simulink model "h_bridge_cascaded_five_level_inverter"  (R2022b)
settings: Solver=ode3  StartTime=0.0  StopTime=0.045  FixedStep=1e-6  RelTol=1e-3  EnableMultiTasking=on
undefined symbols (not defined in the file): fc, fr, Ma, ph
libraries: spsIGBTDiodeLib x328, simulink x164, spsDCVoltageSourceLib x82, spsCurrentMeasurementLib x41, spsSeriesRLCBranchLib x41, spsVoltageMeasurementLib x41, spspowerguiLib x1
(part 3 of 3)

== system h_bridge_cascaded_five_level_inverter/Phase A33 ==
  100V : spsDCVoltageSourceLib/DC Voltage Source  Amplitude=100  Measurements=None
  100V1 : spsDCVoltageSourceLib/DC Voltage Source  Amplitude=100  Measurements=None
  NOT{,1..3} (4 alike) : Logic  Operator=NOT  AllPortsSameDT=off  OutDataTypeStr=boolean
  Relational Operator4 : RelationalOperator  OutDataTypeStr=boolean  InputSameDT=off
  Relational Operator5 : RelationalOperator  Operator=<=  OutDataTypeStr=boolean  InputSameDT=off
  Relational Operator6 : RelationalOperator  Operator=<=  OutDataTypeStr=boolean  InputSameDT=off
  Relational Operator7 : RelationalOperator  OutDataTypeStr=boolean  InputSameDT=off
  Repeating Sequence1 : simulink/Sources/Repeating Sequence  rep_seq_t=[0 0.00025 0.0005 0.00075 0.001]*(1/fr)*(1/fc)*(1/2)  rep_seq_y="[0 1 0 -1 0  ]"
  Repeating Sequence2 : simulink/Sources/Repeating Sequence  rep_seq_t=[0 0.00025 0.0005 0.00075 0.001]*(1/fr)*(1/fc)*(1/2)  rep_seq_y=[ 0 -1 0 1 0 ]
  Repeating Sequence5 : simulink/Sources/Repeating Sequence  rep_seq_t=[0 0.00025 0.0005 0.00075 0.001]*(1/fr)*(1/fc)*(1/2)  rep_seq_y=[1 0 -1 0 1]
  Repeating Sequence7 : simulink/Sources/Repeating Sequence  rep_seq_t=[0 0.00025 0.0005 0.00075 0.001]*(1/fr)*(1/fc)*(1/2)  rep_seq_y=[-1 0 1 0 -1]
  SW{1..8} (8 alike) : spsIGBTDiodeLib/IGBT//Diode  Ron=1e-3  Rs=1e5  Cs=inf  Measurements=on
  Sine Wave1 : Sin  Amplitude=Ma  Frequency=2*pi*fr  Phase=ph  SampleTime=0
  Sine Wave2 : Sin  Amplitude=Ma  Frequency=2*pi*fr  Phase=ph  SampleTime=0
  Va : PMIOPort  Tag=PMCPort  Side=Right
  N : PMIOPort  Tag=PMCPort  Port=2  Side=Right
  wires:
  Sine Wave2/1 -> Relational Operator4/1, Relational Operator6/1
  Repeating Sequence1/1 -> Relational Operator4/2
  Repeating Sequence2/1 -> Relational Operator6/2
  Relational Operator4/1 -> NOT/1, [S1]
  NOT/1 -> [S3]
  NOT1/1 -> [S4]
  Relational Operator6/1 -> [S2], NOT1/1
  Repeating Sequence7/1 -> Relational Operator7/2
  Repeating Sequence5/1 -> Relational Operator5/2
  Sine Wave1/1 -> Relational Operator7/1, Relational Operator5/1
  Relational Operator5/1 -> [S6], NOT3/1
  Relational Operator7/1 -> [S5], NOT2/1
  NOT2/1 -> [S7]
  NOT3/1 -> [S8]
  [S3] -> SW3/1
  [S6] -> SW6/1
  [S8] -> SW8/1
  [S1] -> SW1/1
  [S2] -> SW2/1
  [S4] -> SW4/1
  [S5] -> SW5/1
  connections:
  Va/RConn1 -- SW2/RConn1 -- SW4/LConn1
  SW4/RConn1 -- 100V/LConn1 -- SW3/RConn1
  SW8/RConn1 -- 100V1/LConn1 -- SW7/RConn1
  SW1/RConn1 -- SW3/LConn1 -- SW6/RConn1 -- SW8/LConn1
  SW5/LConn1 -- 100V1/RConn1 -- SW6/LConn1
  N/RConn1 -- SW5/RConn1 -- SW7/LConn1
  100V/RConn1 -- SW1/LConn1 -- SW2/LConn1

== system h_bridge_cascaded_five_level_inverter/Phase A34 ==
  100V : spsDCVoltageSourceLib/DC Voltage Source  Amplitude=100  Measurements=None
  100V1 : spsDCVoltageSourceLib/DC Voltage Source  Amplitude=100  Measurements=None
  NOT{,1..3} (4 alike) : Logic  Operator=NOT  AllPortsSameDT=off  OutDataTypeStr=boolean
  Relational Operator4 : RelationalOperator  OutDataTypeStr=boolean  InputSameDT=off
  Relational Operator5 : RelationalOperator  Operator=<=  OutDataTypeStr=boolean  InputSameDT=off
  Relational Operator6 : RelationalOperator  Operator=<=  OutDataTypeStr=boolean  InputSameDT=off
  Relational Operator7 : RelationalOperator  OutDataTypeStr=boolean  InputSameDT=off
  Repeating Sequence1 : simulink/Sources/Repeating Sequence  rep_seq_t=[0 0.00025 0.0005 0.00075 0.001]*(1/fr)*(1/fc)*(1/2)  rep_seq_y="[0 1 0 -1 0  ]"
  Repeating Sequence2 : simulink/Sources/Repeating Sequence  rep_seq_t=[0 0.00025 0.0005 0.00075 0.001]*(1/fr)*(1/fc)*(1/2)  rep_seq_y=[ 0 -1 0 1 0 ]
  Repeating Sequence5 : simulink/Sources/Repeating Sequence  rep_seq_t=[0 0.00025 0.0005 0.00075 0.001]*(1/fr)*(1/fc)*(1/2)  rep_seq_y=[1 0 -1 0 1]
  Repeating Sequence7 : simulink/Sources/Repeating Sequence  rep_seq_t=[0 0.00025 0.0005 0.00075 0.001]*(1/fr)*(1/fc)*(1/2)  rep_seq_y=[-1 0 1 0 -1]
  SW{1..8} (8 alike) : spsIGBTDiodeLib/IGBT//Diode  Ron=1e-3  Rs=1e5  Cs=inf  Measurements=on
  Sine Wave1 : Sin  Amplitude=Ma  Frequency=2*pi*fr  Phase=ph  SampleTime=0
  Sine Wave2 : Sin  Amplitude=Ma  Frequency=2*pi*fr  Phase=ph  SampleTime=0
  Va : PMIOPort  Tag=PMCPort  Side=Right
  N : PMIOPort  Tag=PMCPort  Port=2  Side=Right
  wires:
  Sine Wave2/1 -> Relational Operator4/1, Relational Operator6/1
  Repeating Sequence1/1 -> Relational Operator4/2
  Repeating Sequence2/1 -> Relational Operator6/2
  Relational Operator4/1 -> NOT/1, [S1]
  NOT/1 -> [S3]
  NOT1/1 -> [S4]
  Relational Operator6/1 -> [S2], NOT1/1
  Repeating Sequence7/1 -> Relational Operator7/2
  Repeating Sequence5/1 -> Relational Operator5/2
  Sine Wave1/1 -> Relational Operator7/1, Relational Operator5/1
  Relational Operator5/1 -> [S6], NOT3/1
  Relational Operator7/1 -> [S5], NOT2/1
  NOT2/1 -> [S7]
  NOT3/1 -> [S8]
  [S3] -> SW3/1
  [S6] -> SW6/1
  [S7] -> SW7/1
  [S8] -> SW8/1
  [S1] -> SW1/1
  [S2] -> SW2/1
  [S4] -> SW4/1
  connections:
  Va/RConn1 -- SW2/RConn1 -- SW4/LConn1
  SW4/RConn1 -- 100V/LConn1 -- SW3/RConn1
  SW8/RConn1 -- 100V1/LConn1 -- SW7/RConn1
  SW1/RConn1 -- SW3/LConn1 -- SW6/RConn1 -- SW8/LConn1
  SW5/LConn1 -- 100V1/RConn1 -- SW6/LConn1
  N/RConn1 -- SW5/RConn1 -- SW7/LConn1
  100V/RConn1 -- SW1/LConn1 -- SW2/LConn1

== system h_bridge_cascaded_five_level_inverter/Phase A42 ==
  100V : spsDCVoltageSourceLib/DC Voltage Source  Amplitude=100  Measurements=None
  100V1 : spsDCVoltageSourceLib/DC Voltage Source  Amplitude=100  Measurements=None
  NOT{,1..3} (4 alike) : Logic  Operator=NOT  AllPortsSameDT=off  OutDataTypeStr=boolean
  Relational Operator4 : RelationalOperator  OutDataTypeStr=boolean  InputSameDT=off
  Relational Operator5 : RelationalOperator  Operator=<=  OutDataTypeStr=boolean  InputSameDT=off
  Relational Operator6 : RelationalOperator  Operator=<=  OutDataTypeStr=boolean  InputSameDT=off
  Relational Operator7 : RelationalOperator  OutDataTypeStr=boolean  InputSameDT=off
  Repeating Sequence1 : simulink/Sources/Repeating Sequence  rep_seq_t=[0 0.00025 0.0005 0.00075 0.001]*(1/fr)*(1/fc)*(1/2)  rep_seq_y="[0 1 0 -1 0  ]"
  Repeating Sequence2 : simulink/Sources/Repeating Sequence  rep_seq_t=[0 0.00025 0.0005 0.00075 0.001]*(1/fr)*(1/fc)*(1/2)  rep_seq_y=[ 0 -1 0 1 0 ]
  Repeating Sequence5 : simulink/Sources/Repeating Sequence  rep_seq_t=[0 0.00025 0.0005 0.00075 0.001]*(1/fr)*(1/fc)*(1/2)  rep_seq_y=[1 0 -1 0 1]
  Repeating Sequence7 : simulink/Sources/Repeating Sequence  rep_seq_t=[0 0.00025 0.0005 0.00075 0.001]*(1/fr)*(1/fc)*(1/2)  rep_seq_y=[-1 0 1 0 -1]
  SW{1,3..8} (7 alike) : spsIGBTDiodeLib/IGBT//Diode  Ron=1e-3  Rs=1e5  Cs=inf  Measurements=on
  SW2 : spsIGBTDiodeLib/IGBT//Diode  Ron=f5_internal_r  Rs=1e5  Cs=inf  Measurements=on
  Sine Wave1 : Sin  Amplitude=Ma  Frequency=2*pi*fr  Phase=ph  SampleTime=0
  Sine Wave2 : Sin  Amplitude=Ma  Frequency=2*pi*fr  Phase=ph  SampleTime=0
  Va : PMIOPort  Tag=PMCPort  Side=Right
  N : PMIOPort  Tag=PMCPort  Port=2  Side=Right
  wires:
  Sine Wave2/1 -> Relational Operator4/1, Relational Operator6/1
  Repeating Sequence1/1 -> Relational Operator4/2
  Repeating Sequence2/1 -> Relational Operator6/2
  Relational Operator4/1 -> NOT/1, [S1]
  NOT/1 -> [S3]
  NOT1/1 -> [S4]
  Relational Operator6/1 -> [S2], NOT1/1
  Repeating Sequence7/1 -> Relational Operator7/2
  Repeating Sequence5/1 -> Relational Operator5/2
  Sine Wave1/1 -> Relational Operator7/1, Relational Operator5/1
  Relational Operator5/1 -> [S6], NOT3/1
  Relational Operator7/1 -> [S5], NOT2/1
  NOT2/1 -> [S7]
  NOT3/1 -> [S8]
  [S3] -> SW3/1
  [S4] -> SW4/1
  [S6] -> SW6/1
  [S5] -> SW5/1
  [S7] -> SW7/1
  [S8] -> SW8/1
  [S1] -> SW1/1
  [S2] -> SW2/1
  connections:
  Va/RConn1 -- SW2/RConn1 -- SW4/LConn1
  SW4/RConn1 -- 100V/LConn1 -- SW3/RConn1
  SW8/RConn1 -- 100V1/LConn1 -- SW7/RConn1
  SW1/RConn1 -- SW3/LConn1 -- SW6/RConn1 -- SW8/LConn1
  SW5/LConn1 -- 100V1/RConn1 -- SW6/LConn1
  N/RConn1 -- SW5/RConn1 -- SW7/LConn1
  100V/RConn1 -- SW1/LConn1 -- SW2/LConn1

== system h_bridge_cascaded_five_level_inverter/Phase A43 ==
  100V : spsDCVoltageSourceLib/DC Voltage Source  Amplitude=100  Measurements=None
  100V1 : spsDCVoltageSourceLib/DC Voltage Source  Amplitude=100  Measurements=None
  NOT{,1..3} (4 alike) : Logic  Operator=NOT  AllPortsSameDT=off  OutDataTypeStr=boolean
  Relational Operator4 : RelationalOperator  OutDataTypeStr=boolean  InputSameDT=off
  Relational Operator5 : RelationalOperator  Operator=<=  OutDataTypeStr=boolean  InputSameDT=off
  Relational Operator6 : RelationalOperator  Operator=<=  OutDataTypeStr=boolean  InputSameDT=off
  Relational Operator7 : RelationalOperator  OutDataTypeStr=boolean  InputSameDT=off
  Repeating Sequence1 : simulink/Sources/Repeating Sequence  rep_seq_t=[0 0.00025 0.0005 0.00075 0.001]*(1/fr)*(1/fc)*(1/2)  rep_seq_y="[0 1 0 -1 0  ]"
  Repeating Sequence2 : simulink/Sources/Repeating Sequence  rep_seq_t=[0 0.00025 0.0005 0.00075 0.001]*(1/fr)*(1/fc)*(1/2)  rep_seq_y=[ 0 -1 0 1 0 ]
  Repeating Sequence5 : simulink/Sources/Repeating Sequence  rep_seq_t=[0 0.00025 0.0005 0.00075 0.001]*(1/fr)*(1/fc)*(1/2)  rep_seq_y=[1 0 -1 0 1]
  Repeating Sequence7 : simulink/Sources/Repeating Sequence  rep_seq_t=[0 0.00025 0.0005 0.00075 0.001]*(1/fr)*(1/fc)*(1/2)  rep_seq_y=[-1 0 1 0 -1]
  SW{1..3,5..8} (7 alike) : spsIGBTDiodeLib/IGBT//Diode  Ron=1e-3  Rs=1e5  Cs=inf  Measurements=on
  SW4 : spsIGBTDiodeLib/IGBT//Diode  Ron=f5_internal_r  Rs=1e5  Cs=inf  Measurements=on
  Sine Wave1 : Sin  Amplitude=Ma  Frequency=2*pi*fr  Phase=ph  SampleTime=0
  Sine Wave2 : Sin  Amplitude=Ma  Frequency=2*pi*fr  Phase=ph  SampleTime=0
  Va : PMIOPort  Tag=PMCPort  Side=Right
  N : PMIOPort  Tag=PMCPort  Port=2  Side=Right
  wires:
  Sine Wave2/1 -> Relational Operator4/1, Relational Operator6/1
  Repeating Sequence1/1 -> Relational Operator4/2
  Repeating Sequence2/1 -> Relational Operator6/2
  Relational Operator4/1 -> NOT/1, [S1]
  NOT/1 -> [S3]
  NOT1/1 -> [S4]
  Relational Operator6/1 -> [S2], NOT1/1
  Repeating Sequence7/1 -> Relational Operator7/2
  Repeating Sequence5/1 -> Relational Operator5/2
  Sine Wave1/1 -> Relational Operator7/1, Relational Operator5/1
  Relational Operator5/1 -> [S6], NOT3/1
  Relational Operator7/1 -> [S5], NOT2/1
  NOT2/1 -> [S7]
  NOT3/1 -> [S8]
  [S3] -> SW3/1
  [S4] -> SW4/1
  [S6] -> SW6/1
  [S5] -> SW5/1
  [S7] -> SW7/1
  [S8] -> SW8/1
  [S1] -> SW1/1
  [S2] -> SW2/1
  connections:
  Va/RConn1 -- SW2/RConn1 -- SW4/LConn1
  SW4/RConn1 -- 100V/LConn1 -- SW3/RConn1
  SW8/RConn1 -- 100V1/LConn1 -- SW7/RConn1
  SW1/RConn1 -- SW3/LConn1 -- SW6/RConn1 -- SW8/LConn1
  SW5/LConn1 -- 100V1/RConn1 -- SW6/LConn1
  N/RConn1 -- SW5/RConn1 -- SW7/LConn1
  100V/RConn1 -- SW1/LConn1 -- SW2/LConn1

== system h_bridge_cascaded_five_level_inverter/Phase A44 ==
  100V : spsDCVoltageSourceLib/DC Voltage Source  Amplitude=100  Measurements=None
  100V1 : spsDCVoltageSourceLib/DC Voltage Source  Amplitude=100  Measurements=None
  NOT{,1..3} (4 alike) : Logic  Operator=NOT  AllPortsSameDT=off  OutDataTypeStr=boolean
  Relational Operator4 : RelationalOperator  OutDataTypeStr=boolean  InputSameDT=off
  Relational Operator5 : RelationalOperator  Operator=<=  OutDataTypeStr=boolean  InputSameDT=off
  Relational Operator6 : RelationalOperator  Operator=<=  OutDataTypeStr=boolean  InputSameDT=off
  Relational Operator7 : RelationalOperator  OutDataTypeStr=boolean  InputSameDT=off
  Repeating Sequence1 : simulink/Sources/Repeating Sequence  rep_seq_t=[0 0.00025 0.0005 0.00075 0.001]*(1/fr)*(1/fc)*(1/2)  rep_seq_y="[0 1 0 -1 0  ]"
  Repeating Sequence2 : simulink/Sources/Repeating Sequence  rep_seq_t=[0 0.00025 0.0005 0.00075 0.001]*(1/fr)*(1/fc)*(1/2)  rep_seq_y=[ 0 -1 0 1 0 ]
  Repeating Sequence5 : simulink/Sources/Repeating Sequence  rep_seq_t=[0 0.00025 0.0005 0.00075 0.001]*(1/fr)*(1/fc)*(1/2)  rep_seq_y=[1 0 -1 0 1]
  Repeating Sequence7 : simulink/Sources/Repeating Sequence  rep_seq_t=[0 0.00025 0.0005 0.00075 0.001]*(1/fr)*(1/fc)*(1/2)  rep_seq_y=[-1 0 1 0 -1]
  SW{1..2,4..8} (7 alike) : spsIGBTDiodeLib/IGBT//Diode  Ron=1e-3  Rs=1e5  Cs=inf  Measurements=on
  SW3 : spsIGBTDiodeLib/IGBT//Diode  Ron=f5_internal_r  Rs=1e5  Cs=inf  Measurements=on
  Sine Wave1 : Sin  Amplitude=Ma  Frequency=2*pi*fr  Phase=ph  SampleTime=0
  Sine Wave2 : Sin  Amplitude=Ma  Frequency=2*pi*fr  Phase=ph  SampleTime=0
  Va : PMIOPort  Tag=PMCPort  Side=Right
  N : PMIOPort  Tag=PMCPort  Port=2  Side=Right
  wires:
  Sine Wave2/1 -> Relational Operator4/1, Relational Operator6/1
  Repeating Sequence1/1 -> Relational Operator4/2
  Repeating Sequence2/1 -> Relational Operator6/2
  Relational Operator4/1 -> NOT/1, [S1]
  NOT/1 -> [S3]
  NOT1/1 -> [S4]
  Relational Operator6/1 -> [S2], NOT1/1
  Repeating Sequence7/1 -> Relational Operator7/2
  Repeating Sequence5/1 -> Relational Operator5/2
  Sine Wave1/1 -> Relational Operator7/1, Relational Operator5/1
  Relational Operator5/1 -> [S6], NOT3/1
  Relational Operator7/1 -> [S5], NOT2/1
  NOT2/1 -> [S7]
  NOT3/1 -> [S8]
  [S3] -> SW3/1
  [S4] -> SW4/1
  [S6] -> SW6/1
  [S5] -> SW5/1
  [S7] -> SW7/1
  [S8] -> SW8/1
  [S1] -> SW1/1
  [S2] -> SW2/1
  connections:
  Va/RConn1 -- SW2/RConn1 -- SW4/LConn1
  SW4/RConn1 -- 100V/LConn1 -- SW3/RConn1
  SW8/RConn1 -- 100V1/LConn1 -- SW7/RConn1
  SW1/RConn1 -- SW3/LConn1 -- SW6/RConn1 -- SW8/LConn1
  SW5/LConn1 -- 100V1/RConn1 -- SW6/LConn1
  N/RConn1 -- SW5/RConn1 -- SW7/LConn1
  100V/RConn1 -- SW1/LConn1 -- SW2/LConn1

== system h_bridge_cascaded_five_level_inverter/Phase A45 ==
  100V : spsDCVoltageSourceLib/DC Voltage Source  Amplitude=100  Measurements=None
  100V1 : spsDCVoltageSourceLib/DC Voltage Source  Amplitude=100  Measurements=None
  NOT{,1..3} (4 alike) : Logic  Operator=NOT  AllPortsSameDT=off  OutDataTypeStr=boolean
  Relational Operator4 : RelationalOperator  OutDataTypeStr=boolean  InputSameDT=off
  Relational Operator5 : RelationalOperator  Operator=<=  OutDataTypeStr=boolean  InputSameDT=off
  Relational Operator6 : RelationalOperator  Operator=<=  OutDataTypeStr=boolean  InputSameDT=off
  Relational Operator7 : RelationalOperator  OutDataTypeStr=boolean  InputSameDT=off
  Repeating Sequence1 : simulink/Sources/Repeating Sequence  rep_seq_t=[0 0.00025 0.0005 0.00075 0.001]*(1/fr)*(1/fc)*(1/2)  rep_seq_y="[0 1 0 -1 0  ]"
  Repeating Sequence2 : simulink/Sources/Repeating Sequence  rep_seq_t=[0 0.00025 0.0005 0.00075 0.001]*(1/fr)*(1/fc)*(1/2)  rep_seq_y=[ 0 -1 0 1 0 ]
  Repeating Sequence5 : simulink/Sources/Repeating Sequence  rep_seq_t=[0 0.00025 0.0005 0.00075 0.001]*(1/fr)*(1/fc)*(1/2)  rep_seq_y=[1 0 -1 0 1]
  Repeating Sequence7 : simulink/Sources/Repeating Sequence  rep_seq_t=[0 0.00025 0.0005 0.00075 0.001]*(1/fr)*(1/fc)*(1/2)  rep_seq_y=[-1 0 1 0 -1]
  SW{1..5,7..8} (7 alike) : spsIGBTDiodeLib/IGBT//Diode  Ron=1e-3  Rs=1e5  Cs=inf  Measurements=on
  SW6 : spsIGBTDiodeLib/IGBT//Diode  Ron=f5_internal_r  Rs=1e5  Cs=inf  Measurements=on
  Sine Wave1 : Sin  Amplitude=Ma  Frequency=2*pi*fr  Phase=ph  SampleTime=0
  Sine Wave2 : Sin  Amplitude=Ma  Frequency=2*pi*fr  Phase=ph  SampleTime=0
  Va : PMIOPort  Tag=PMCPort  Side=Right
  N : PMIOPort  Tag=PMCPort  Port=2  Side=Right
  wires:
  Sine Wave2/1 -> Relational Operator4/1, Relational Operator6/1
  Repeating Sequence1/1 -> Relational Operator4/2
  Repeating Sequence2/1 -> Relational Operator6/2
  Relational Operator4/1 -> NOT/1, [S1]
  NOT/1 -> [S3]
  NOT1/1 -> [S4]
  Relational Operator6/1 -> [S2], NOT1/1
  Repeating Sequence7/1 -> Relational Operator7/2
  Repeating Sequence5/1 -> Relational Operator5/2
  Sine Wave1/1 -> Relational Operator7/1, Relational Operator5/1
  Relational Operator5/1 -> [S6], NOT3/1
  Relational Operator7/1 -> [S5], NOT2/1
  NOT2/1 -> [S7]
  NOT3/1 -> [S8]
  [S3] -> SW3/1
  [S4] -> SW4/1
  [S6] -> SW6/1
  [S5] -> SW5/1
  [S7] -> SW7/1
  [S8] -> SW8/1
  [S1] -> SW1/1
  [S2] -> SW2/1
  connections:
  Va/RConn1 -- SW2/RConn1 -- SW4/LConn1
  SW4/RConn1 -- 100V/LConn1 -- SW3/RConn1
  SW8/RConn1 -- 100V1/LConn1 -- SW7/RConn1
  SW1/RConn1 -- SW3/LConn1 -- SW6/RConn1 -- SW8/LConn1
  SW5/LConn1 -- 100V1/RConn1 -- SW6/LConn1
  N/RConn1 -- SW5/RConn1 -- SW7/LConn1
  100V/RConn1 -- SW1/LConn1 -- SW2/LConn1

== system h_bridge_cascaded_five_level_inverter/Phase A46 ==
  100V : spsDCVoltageSourceLib/DC Voltage Source  Amplitude=100  Measurements=None
  100V1 : spsDCVoltageSourceLib/DC Voltage Source  Amplitude=100  Measurements=None
  NOT{,1..3} (4 alike) : Logic  Operator=NOT  AllPortsSameDT=off  OutDataTypeStr=boolean
  Relational Operator4 : RelationalOperator  OutDataTypeStr=boolean  InputSameDT=off
  Relational Operator5 : RelationalOperator  Operator=<=  OutDataTypeStr=boolean  InputSameDT=off
  Relational Operator6 : RelationalOperator  Operator=<=  OutDataTypeStr=boolean  InputSameDT=off
  Relational Operator7 : RelationalOperator  OutDataTypeStr=boolean  InputSameDT=off
  Repeating Sequence1 : simulink/Sources/Repeating Sequence  rep_seq_t=[0 0.00025 0.0005 0.00075 0.001]*(1/fr)*(1/fc)*(1/2)  rep_seq_y="[0 1 0 -1 0  ]"
  Repeating Sequence2 : simulink/Sources/Repeating Sequence  rep_seq_t=[0 0.00025 0.0005 0.00075 0.001]*(1/fr)*(1/fc)*(1/2)  rep_seq_y=[ 0 -1 0 1 0 ]
  Repeating Sequence5 : simulink/Sources/Repeating Sequence  rep_seq_t=[0 0.00025 0.0005 0.00075 0.001]*(1/fr)*(1/fc)*(1/2)  rep_seq_y=[1 0 -1 0 1]
  Repeating Sequence7 : simulink/Sources/Repeating Sequence  rep_seq_t=[0 0.00025 0.0005 0.00075 0.001]*(1/fr)*(1/fc)*(1/2)  rep_seq_y=[-1 0 1 0 -1]
  SW{1..7} (7 alike) : spsIGBTDiodeLib/IGBT//Diode  Ron=1e-3  Rs=1e5  Cs=inf  Measurements=on
  SW8 : spsIGBTDiodeLib/IGBT//Diode  Ron=f5_internal_r  Rs=1e5  Cs=inf  Measurements=on
  Sine Wave1 : Sin  Amplitude=Ma  Frequency=2*pi*fr  Phase=ph  SampleTime=0
  Sine Wave2 : Sin  Amplitude=Ma  Frequency=2*pi*fr  Phase=ph  SampleTime=0
  Va : PMIOPort  Tag=PMCPort  Side=Right
  N : PMIOPort  Tag=PMCPort  Port=2  Side=Right
  wires:
  Sine Wave2/1 -> Relational Operator4/1, Relational Operator6/1
  Repeating Sequence1/1 -> Relational Operator4/2
  Repeating Sequence2/1 -> Relational Operator6/2
  Relational Operator4/1 -> NOT/1, [S1]
  NOT/1 -> [S3]
  NOT1/1 -> [S4]
  Relational Operator6/1 -> [S2], NOT1/1
  Repeating Sequence7/1 -> Relational Operator7/2
  Repeating Sequence5/1 -> Relational Operator5/2
  Sine Wave1/1 -> Relational Operator7/1, Relational Operator5/1
  Relational Operator5/1 -> [S6], NOT3/1
  Relational Operator7/1 -> [S5], NOT2/1
  NOT2/1 -> [S7]
  NOT3/1 -> [S8]
  [S3] -> SW3/1
  [S4] -> SW4/1
  [S6] -> SW6/1
  [S5] -> SW5/1
  [S7] -> SW7/1
  [S8] -> SW8/1
  [S1] -> SW1/1
  [S2] -> SW2/1
  connections:
  Va/RConn1 -- SW2/RConn1 -- SW4/LConn1
  SW4/RConn1 -- 100V/LConn1 -- SW3/RConn1
  SW8/RConn1 -- 100V1/LConn1 -- SW7/RConn1
  SW1/RConn1 -- SW3/LConn1 -- SW6/RConn1 -- SW8/LConn1
  SW5/LConn1 -- 100V1/RConn1 -- SW6/LConn1
  N/RConn1 -- SW5/RConn1 -- SW7/LConn1
  100V/RConn1 -- SW1/LConn1 -- SW2/LConn1

== system h_bridge_cascaded_five_level_inverter/Phase A47 ==
  100V : spsDCVoltageSourceLib/DC Voltage Source  Amplitude=100  Measurements=None
  100V1 : spsDCVoltageSourceLib/DC Voltage Source  Amplitude=100  Measurements=None
  NOT{,1..3} (4 alike) : Logic  Operator=NOT  AllPortsSameDT=off  OutDataTypeStr=boolean
  Relational Operator4 : RelationalOperator  OutDataTypeStr=boolean  InputSameDT=off
  Relational Operator5 : RelationalOperator  Operator=<=  OutDataTypeStr=boolean  InputSameDT=off
  Relational Operator6 : RelationalOperator  Operator=<=  OutDataTypeStr=boolean  InputSameDT=off
  Relational Operator7 : RelationalOperator  OutDataTypeStr=boolean  InputSameDT=off
  Repeating Sequence1 : simulink/Sources/Repeating Sequence  rep_seq_t=[0 0.00025 0.0005 0.00075 0.001]*(1/fr)*(1/fc)*(1/2)  rep_seq_y="[0 1 0 -1 0  ]"
  Repeating Sequence2 : simulink/Sources/Repeating Sequence  rep_seq_t=[0 0.00025 0.0005 0.00075 0.001]*(1/fr)*(1/fc)*(1/2)  rep_seq_y=[ 0 -1 0 1 0 ]
  Repeating Sequence5 : simulink/Sources/Repeating Sequence  rep_seq_t=[0 0.00025 0.0005 0.00075 0.001]*(1/fr)*(1/fc)*(1/2)  rep_seq_y=[1 0 -1 0 1]
  Repeating Sequence7 : simulink/Sources/Repeating Sequence  rep_seq_t=[0 0.00025 0.0005 0.00075 0.001]*(1/fr)*(1/fc)*(1/2)  rep_seq_y=[-1 0 1 0 -1]
  SW{1..6,8} (7 alike) : spsIGBTDiodeLib/IGBT//Diode  Ron=1e-3  Rs=1e5  Cs=inf  Measurements=on
  SW7 : spsIGBTDiodeLib/IGBT//Diode  Ron=f5_internal_r  Rs=1e5  Cs=inf  Measurements=on
  Sine Wave1 : Sin  Amplitude=Ma  Frequency=2*pi*fr  Phase=ph  SampleTime=0
  Sine Wave2 : Sin  Amplitude=Ma  Frequency=2*pi*fr  Phase=ph  SampleTime=0
  Va : PMIOPort  Tag=PMCPort  Side=Right
  N : PMIOPort  Tag=PMCPort  Port=2  Side=Right
  wires:
  Sine Wave2/1 -> Relational Operator4/1, Relational Operator6/1
  Repeating Sequence1/1 -> Relational Operator4/2
  Repeating Sequence2/1 -> Relational Operator6/2
  Relational Operator4/1 -> NOT/1, [S1]
  NOT/1 -> [S3]
  NOT1/1 -> [S4]
  Relational Operator6/1 -> [S2], NOT1/1
  Repeating Sequence7/1 -> Relational Operator7/2
  Repeating Sequence5/1 -> Relational Operator5/2
  Sine Wave1/1 -> Relational Operator7/1, Relational Operator5/1
  Relational Operator5/1 -> [S6], NOT3/1
  Relational Operator7/1 -> [S5], NOT2/1
  NOT2/1 -> [S7]
  NOT3/1 -> [S8]
  [S3] -> SW3/1
  [S4] -> SW4/1
  [S6] -> SW6/1
  [S5] -> SW5/1
  [S7] -> SW7/1
  [S8] -> SW8/1
  [S1] -> SW1/1
  [S2] -> SW2/1
  connections:
  Va/RConn1 -- SW2/RConn1 -- SW4/LConn1
  SW4/RConn1 -- 100V/LConn1 -- SW3/RConn1
  SW8/RConn1 -- 100V1/LConn1 -- SW7/RConn1
  SW1/RConn1 -- SW3/LConn1 -- SW6/RConn1 -- SW8/LConn1
  SW5/LConn1 -- 100V1/RConn1 -- SW6/LConn1
  N/RConn1 -- SW5/RConn1 -- SW7/LConn1
  100V/RConn1 -- SW1/LConn1 -- SW2/LConn1

== system h_bridge_cascaded_five_level_inverter/Phase A48 ==
  100V : spsDCVoltageSourceLib/DC Voltage Source  Amplitude=100  Measurements=None
  100V1 : spsDCVoltageSourceLib/DC Voltage Source  Amplitude=100  Measurements=None
  NOT{,1..3} (4 alike) : Logic  Operator=NOT  AllPortsSameDT=off  OutDataTypeStr=boolean
  Relational Operator4 : RelationalOperator  OutDataTypeStr=boolean  InputSameDT=off
  Relational Operator5 : RelationalOperator  Operator=<=  OutDataTypeStr=boolean  InputSameDT=off
  Relational Operator6 : RelationalOperator  Operator=<=  OutDataTypeStr=boolean  InputSameDT=off
  Relational Operator7 : RelationalOperator  OutDataTypeStr=boolean  InputSameDT=off
  Repeating Sequence1 : simulink/Sources/Repeating Sequence  rep_seq_t=[0 0.00025 0.0005 0.00075 0.001]*(1/fr)*(1/fc)*(1/2)  rep_seq_y="[0 1 0 -1 0  ]"
  Repeating Sequence2 : simulink/Sources/Repeating Sequence  rep_seq_t=[0 0.00025 0.0005 0.00075 0.001]*(1/fr)*(1/fc)*(1/2)  rep_seq_y=[ 0 -1 0 1 0 ]
  Repeating Sequence5 : simulink/Sources/Repeating Sequence  rep_seq_t=[0 0.00025 0.0005 0.00075 0.001]*(1/fr)*(1/fc)*(1/2)  rep_seq_y=[1 0 -1 0 1]
  Repeating Sequence7 : simulink/Sources/Repeating Sequence  rep_seq_t=[0 0.00025 0.0005 0.00075 0.001]*(1/fr)*(1/fc)*(1/2)  rep_seq_y=[-1 0 1 0 -1]
  SW{1..4,6..8} (7 alike) : spsIGBTDiodeLib/IGBT//Diode  Ron=1e-3  Rs=1e5  Cs=inf  Measurements=on
  SW5 : spsIGBTDiodeLib/IGBT//Diode  Ron=f5_internal_r  Rs=1e5  Cs=inf  Measurements=on
  Sine Wave1 : Sin  Amplitude=Ma  Frequency=2*pi*fr  Phase=ph  SampleTime=0
  Sine Wave2 : Sin  Amplitude=Ma  Frequency=2*pi*fr  Phase=ph  SampleTime=0
  Va : PMIOPort  Tag=PMCPort  Side=Right
  N : PMIOPort  Tag=PMCPort  Port=2  Side=Right
  wires:
  Sine Wave2/1 -> Relational Operator4/1, Relational Operator6/1
  Repeating Sequence1/1 -> Relational Operator4/2
  Repeating Sequence2/1 -> Relational Operator6/2
  Relational Operator4/1 -> NOT/1, [S1]
  NOT/1 -> [S3]
  NOT1/1 -> [S4]
  Relational Operator6/1 -> [S2], NOT1/1
  Repeating Sequence7/1 -> Relational Operator7/2
  Repeating Sequence5/1 -> Relational Operator5/2
  Sine Wave1/1 -> Relational Operator7/1, Relational Operator5/1
  Relational Operator5/1 -> [S6], NOT3/1
  Relational Operator7/1 -> [S5], NOT2/1
  NOT2/1 -> [S7]
  NOT3/1 -> [S8]
  [S3] -> SW3/1
  [S4] -> SW4/1
  [S6] -> SW6/1
  [S5] -> SW5/1
  [S7] -> SW7/1
  [S8] -> SW8/1
  [S1] -> SW1/1
  [S2] -> SW2/1
  connections:
  Va/RConn1 -- SW2/RConn1 -- SW4/LConn1
  SW4/RConn1 -- 100V/LConn1 -- SW3/RConn1
  SW8/RConn1 -- 100V1/LConn1 -- SW7/RConn1
  SW1/RConn1 -- SW3/LConn1 -- SW6/RConn1 -- SW8/LConn1
  SW5/LConn1 -- 100V1/RConn1 -- SW6/LConn1
  N/RConn1 -- SW5/RConn1 -- SW7/LConn1
  100V/RConn1 -- SW1/LConn1 -- SW2/LConn1

== system h_bridge_cascaded_five_level_inverter/Phase A5 ==
  100V : spsDCVoltageSourceLib/DC Voltage Source  Amplitude=100  Measurements=None
  100V1 : spsDCVoltageSourceLib/DC Voltage Source  Amplitude=100  Measurements=None
  NOT{,1..3} (4 alike) : Logic  Operator=NOT  AllPortsSameDT=off  OutDataTypeStr=boolean
  Relational Operator4 : RelationalOperator  OutDataTypeStr=boolean  InputSameDT=off
  Relational Operator5 : RelationalOperator  Operator=<=  OutDataTypeStr=boolean  InputSameDT=off
  Relational Operator6 : RelationalOperator  Operator=<=  OutDataTypeStr=boolean  InputSameDT=off
  Relational Operator7 : RelationalOperator  OutDataTypeStr=boolean  InputSameDT=off
  Repeating Sequence1 : simulink/Sources/Repeating Sequence  rep_seq_t=[0 0.00025 0.0005 0.00075 0.001]*(1/fr)*(1/fc)*(1/2)  rep_seq_y="[0 1 0 -1 0  ]"
  Repeating Sequence2 : simulink/Sources/Repeating Sequence  rep_seq_t=[0 0.00025 0.0005 0.00075 0.001]*(1/fr)*(1/fc)*(1/2)  rep_seq_y=[ 0 -1 0 1 0 ]
  Repeating Sequence5 : simulink/Sources/Repeating Sequence  rep_seq_t=[0 0.00025 0.0005 0.00075 0.001]*(1/fr)*(1/fc)*(1/2)  rep_seq_y=[1 0 -1 0 1]
  Repeating Sequence7 : simulink/Sources/Repeating Sequence  rep_seq_t=[0 0.00025 0.0005 0.00075 0.001]*(1/fr)*(1/fc)*(1/2)  rep_seq_y=[-1 0 1 0 -1]
  SW{1..8} (8 alike) : spsIGBTDiodeLib/IGBT//Diode  Ron=1e-3  Rs=1e5  Cs=inf  Measurements=on
  Sine Wave1 : Sin  Amplitude=Ma  Frequency=2*pi*fr  Phase=ph  SampleTime=0
  Sine Wave2 : Sin  Amplitude=Ma  Frequency=2*pi*fr  Phase=ph  SampleTime=0
  Va : PMIOPort  Tag=PMCPort  Side=Right
  N : PMIOPort  Tag=PMCPort  Port=2  Side=Right
  wires:
  Sine Wave2/1 -> Relational Operator4/1, Relational Operator6/1
  Repeating Sequence1/1 -> Relational Operator4/2
  Repeating Sequence2/1 -> Relational Operator6/2
  Relational Operator4/1 -> NOT/1, [S1]
  NOT/1 -> [S3]
  NOT1/1 -> [S4]
  Relational Operator6/1 -> [S2], NOT1/1
  Repeating Sequence7/1 -> Relational Operator7/2
  Repeating Sequence5/1 -> Relational Operator5/2
  Sine Wave1/1 -> Relational Operator7/1, Relational Operator5/1
  Relational Operator5/1 -> [S6], NOT3/1
  Relational Operator7/1 -> [S5], NOT2/1
  NOT2/1 -> [S7]
  NOT3/1 -> [S8]
  [S3] -> SW3/1
  [S6] -> SW6/1
  [S5] -> SW5/1
  [S7] -> SW7/1
  [S8] -> SW8/1
  [S2] -> SW2/1
  [S4] -> SW4/1
  connections:
  Va/RConn1 -- SW2/RConn1 -- SW4/LConn1
  SW4/RConn1 -- 100V/LConn1 -- SW3/RConn1
  SW8/RConn1 -- 100V1/LConn1 -- SW7/RConn1
  SW1/RConn1 -- SW3/LConn1 -- SW6/RConn1 -- SW8/LConn1
  SW5/LConn1 -- 100V1/RConn1 -- SW6/LConn1
  N/RConn1 -- SW5/RConn1 -- SW7/LConn1
  100V/RConn1 -- SW1/LConn1 -- SW2/LConn1

== system h_bridge_cascaded_five_level_inverter/Phase A6 ==
  100V : spsDCVoltageSourceLib/DC Voltage Source  Amplitude=100  Measurements=None
  100V1 : spsDCVoltageSourceLib/DC Voltage Source  Amplitude=100  Measurements=None
  NOT{,1..3} (4 alike) : Logic  Operator=NOT  AllPortsSameDT=off  OutDataTypeStr=boolean
  Relational Operator4 : RelationalOperator  OutDataTypeStr=boolean  InputSameDT=off
  Relational Operator5 : RelationalOperator  Operator=<=  OutDataTypeStr=boolean  InputSameDT=off
  Relational Operator6 : RelationalOperator  Operator=<=  OutDataTypeStr=boolean  InputSameDT=off
  Relational Operator7 : RelationalOperator  OutDataTypeStr=boolean  InputSameDT=off
  Repeating Sequence1 : simulink/Sources/Repeating Sequence  rep_seq_t=[0 0.00025 0.0005 0.00075 0.001]*(1/fr)*(1/fc)*(1/2)  rep_seq_y="[0 1 0 -1 0  ]"
  Repeating Sequence2 : simulink/Sources/Repeating Sequence  rep_seq_t=[0 0.00025 0.0005 0.00075 0.001]*(1/fr)*(1/fc)*(1/2)  rep_seq_y=[ 0 -1 0 1 0 ]
  Repeating Sequence5 : simulink/Sources/Repeating Sequence  rep_seq_t=[0 0.00025 0.0005 0.00075 0.001]*(1/fr)*(1/fc)*(1/2)  rep_seq_y=[1 0 -1 0 1]
  Repeating Sequence7 : simulink/Sources/Repeating Sequence  rep_seq_t=[0 0.00025 0.0005 0.00075 0.001]*(1/fr)*(1/fc)*(1/2)  rep_seq_y=[-1 0 1 0 -1]
  SW1 : spsIGBTDiodeLib/IGBT//Diode  Ron=f5_internal_r  Rs=1e5  Cs=inf  Measurements=on
  SW{2..8} (7 alike) : spsIGBTDiodeLib/IGBT//Diode  Ron=1e-3  Rs=1e5  Cs=inf  Measurements=on
  Sine Wave1 : Sin  Amplitude=Ma  Frequency=2*pi*fr  Phase=ph  SampleTime=0
  Sine Wave2 : Sin  Amplitude=Ma  Frequency=2*pi*fr  Phase=ph  SampleTime=0
  Va : PMIOPort  Tag=PMCPort  Side=Right
  N : PMIOPort  Tag=PMCPort  Port=2  Side=Right
  wires:
  Sine Wave2/1 -> Relational Operator4/1, Relational Operator6/1
  Repeating Sequence1/1 -> Relational Operator4/2
  Repeating Sequence2/1 -> Relational Operator6/2
  Relational Operator4/1 -> NOT/1, [S1]
  NOT/1 -> [S3]
  NOT1/1 -> [S4]
  Relational Operator6/1 -> [S2], NOT1/1
  Repeating Sequence7/1 -> Relational Operator7/2
  Repeating Sequence5/1 -> Relational Operator5/2
  Sine Wave1/1 -> Relational Operator7/1, Relational Operator5/1
  Relational Operator5/1 -> [S6], NOT3/1
  Relational Operator7/1 -> [S5], NOT2/1
  NOT2/1 -> [S7]
  NOT3/1 -> [S8]
  [S3] -> SW3/1
  [S4] -> SW4/1
  [S6] -> SW6/1
  [S5] -> SW5/1
  [S7] -> SW7/1
  [S8] -> SW8/1
  [S1] -> SW1/1
  [S2] -> SW2/1
  connections:
  Va/RConn1 -- SW2/RConn1 -- SW4/LConn1
  SW4/RConn1 -- 100V/LConn1 -- SW3/RConn1
  SW8/RConn1 -- 100V1/LConn1 -- SW7/RConn1
  SW1/RConn1 -- SW3/LConn1 -- SW6/RConn1 -- SW8/LConn1
  SW5/LConn1 -- 100V1/RConn1 -- SW6/LConn1
  N/RConn1 -- SW5/RConn1 -- SW7/LConn1
  100V/RConn1 -- SW1/LConn1 -- SW2/LConn1

== system h_bridge_cascaded_five_level_inverter/Phase A7 ==
  note: collector open circuit
  100V : spsDCVoltageSourceLib/DC Voltage Source  Amplitude=100  Measurements=None
  100V1 : spsDCVoltageSourceLib/DC Voltage Source  Amplitude=100  Measurements=None
  NOT{,1..3} (4 alike) : Logic  Operator=NOT  AllPortsSameDT=off  OutDataTypeStr=boolean
  Relational Operator4 : RelationalOperator  OutDataTypeStr=boolean  InputSameDT=off
  Relational Operator5 : RelationalOperator  Operator=<=  OutDataTypeStr=boolean  InputSameDT=off
  Relational Operator6 : RelationalOperator  Operator=<=  OutDataTypeStr=boolean  InputSameDT=off
  Relational Operator7 : RelationalOperator  OutDataTypeStr=boolean  InputSameDT=off
  Repeating Sequence1 : simulink/Sources/Repeating Sequence  rep_seq_t=[0 0.00025 0.0005 0.00075 0.001]*(1/fr)*(1/fc)*(1/2)  rep_seq_y="[0 1 0 -1 0  ]"
  Repeating Sequence2 : simulink/Sources/Repeating Sequence  rep_seq_t=[0 0.00025 0.0005 0.00075 0.001]*(1/fr)*(1/fc)*(1/2)  rep_seq_y=[ 0 -1 0 1 0 ]
  Repeating Sequence5 : simulink/Sources/Repeating Sequence  rep_seq_t=[0 0.00025 0.0005 0.00075 0.001]*(1/fr)*(1/fc)*(1/2)  rep_seq_y=[1 0 -1 0 1]
  Repeating Sequence7 : simulink/Sources/Repeating Sequence  rep_seq_t=[0 0.00025 0.0005 0.00075 0.001]*(1/fr)*(1/fc)*(1/2)  rep_seq_y=[-1 0 1 0 -1]
  SW{1..8} (8 alike) : spsIGBTDiodeLib/IGBT//Diode  Ron=1e-3  Rs=1e5  Cs=inf  Measurements=on
  Sine Wave1 : Sin  Amplitude=Ma  Frequency=2*pi*fr  Phase=ph  SampleTime=0
  Sine Wave2 : Sin  Amplitude=Ma  Frequency=2*pi*fr  Phase=ph  SampleTime=0
  Va : PMIOPort  Tag=PMCPort  Side=Right
  N : PMIOPort  Tag=PMCPort  Port=2  Side=Right
  wires:
  Sine Wave2/1 -> Relational Operator4/1, Relational Operator6/1
  Repeating Sequence1/1 -> Relational Operator4/2
  Repeating Sequence2/1 -> Relational Operator6/2
  Relational Operator4/1 -> NOT/1, [S1]
  NOT/1 -> [S3]
  NOT1/1 -> [S4]
  Relational Operator6/1 -> [S2], NOT1/1
  Repeating Sequence7/1 -> Relational Operator7/2
  Repeating Sequence5/1 -> Relational Operator5/2
  Sine Wave1/1 -> Relational Operator7/1, Relational Operator5/1
  Relational Operator5/1 -> [S6], NOT3/1
  Relational Operator7/1 -> [S5], NOT2/1
  NOT2/1 -> [S7]
  NOT3/1 -> [S8]
  [S3] -> SW3/1
  [S4] -> SW4/1
  [S6] -> SW6/1
  [S5] -> SW5/1
  [S7] -> SW7/1
  [S8] -> SW8/1
  [S1] -> SW1/1
  [S2] -> SW2/1
  connections:
  Va/RConn1 -- SW2/RConn1 -- SW4/LConn1
  SW4/RConn1 -- 100V/LConn1 -- SW3/RConn1
  SW8/RConn1 -- 100V1/LConn1 -- SW7/RConn1
  SW1/RConn1 -- SW3/LConn1 -- SW6/RConn1 -- SW8/LConn1
  SW6/LConn1 -- SW5/LConn1 -- 100V1/RConn1
  N/RConn1 -- SW5/RConn1 -- SW7/LConn1
  100V/RConn1 -- SW1/LConn1

== system h_bridge_cascaded_five_level_inverter/Phase A8 ==
  note: collector open circuit
  100V : spsDCVoltageSourceLib/DC Voltage Source  Amplitude=100  Measurements=None
  100V1 : spsDCVoltageSourceLib/DC Voltage Source  Amplitude=100  Measurements=None
  NOT{,1..3} (4 alike) : Logic  Operator=NOT  AllPortsSameDT=off  OutDataTypeStr=boolean
  Relational Operator4 : RelationalOperator  OutDataTypeStr=boolean  InputSameDT=off
  Relational Operator5 : RelationalOperator  Operator=<=  OutDataTypeStr=boolean  InputSameDT=off
  Relational Operator6 : RelationalOperator  Operator=<=  OutDataTypeStr=boolean  InputSameDT=off
  Relational Operator7 : RelationalOperator  OutDataTypeStr=boolean  InputSameDT=off
  Repeating Sequence1 : simulink/Sources/Repeating Sequence  rep_seq_t=[0 0.00025 0.0005 0.00075 0.001]*(1/fr)*(1/fc)*(1/2)  rep_seq_y="[0 1 0 -1 0  ]"
  Repeating Sequence2 : simulink/Sources/Repeating Sequence  rep_seq_t=[0 0.00025 0.0005 0.00075 0.001]*(1/fr)*(1/fc)*(1/2)  rep_seq_y=[ 0 -1 0 1 0 ]
  Repeating Sequence5 : simulink/Sources/Repeating Sequence  rep_seq_t=[0 0.00025 0.0005 0.00075 0.001]*(1/fr)*(1/fc)*(1/2)  rep_seq_y=[1 0 -1 0 1]
  Repeating Sequence7 : simulink/Sources/Repeating Sequence  rep_seq_t=[0 0.00025 0.0005 0.00075 0.001]*(1/fr)*(1/fc)*(1/2)  rep_seq_y=[-1 0 1 0 -1]
  SW{1..8} (8 alike) : spsIGBTDiodeLib/IGBT//Diode  Ron=1e-3  Rs=1e5  Cs=inf  Measurements=on
  Sine Wave1 : Sin  Amplitude=Ma  Frequency=2*pi*fr  Phase=ph  SampleTime=0
  Sine Wave2 : Sin  Amplitude=Ma  Frequency=2*pi*fr  Phase=ph  SampleTime=0
  Va : PMIOPort  Tag=PMCPort  Side=Right
  N : PMIOPort  Tag=PMCPort  Port=2  Side=Right
  wires:
  Sine Wave2/1 -> Relational Operator4/1, Relational Operator6/1
  Repeating Sequence1/1 -> Relational Operator4/2
  Repeating Sequence2/1 -> Relational Operator6/2
  Relational Operator4/1 -> NOT/1, [S1]
  NOT/1 -> [S3]
  NOT1/1 -> [S4]
  Relational Operator6/1 -> [S2], NOT1/1
  Repeating Sequence7/1 -> Relational Operator7/2
  Repeating Sequence5/1 -> Relational Operator5/2
  Sine Wave1/1 -> Relational Operator7/1, Relational Operator5/1
  Relational Operator5/1 -> [S6], NOT3/1
  Relational Operator7/1 -> [S5], NOT2/1
  NOT2/1 -> [S7]
  NOT3/1 -> [S8]
  [S3] -> SW3/1
  [S4] -> SW4/1
  [S6] -> SW6/1
  [S5] -> SW5/1
  [S7] -> SW7/1
  [S8] -> SW8/1
  [S1] -> SW1/1
  [S2] -> SW2/1
  connections:
  Va/RConn1 -- SW2/RConn1 -- SW4/LConn1
  SW4/RConn1 -- 100V/LConn1 -- SW3/RConn1
  SW8/RConn1 -- 100V1/LConn1 -- SW7/RConn1
  SW6/RConn1 -- SW1/RConn1
  SW5/LConn1 -- 100V1/RConn1 -- SW6/LConn1
  N/RConn1 -- SW5/RConn1 -- SW7/LConn1
  100V/RConn1 -- SW1/LConn1 -- SW2/LConn1

== system h_bridge_cascaded_five_level_inverter/Phase A9 ==
  note: collector open circuit
  100V : spsDCVoltageSourceLib/DC Voltage Source  Amplitude=100  Measurements=None
  100V1 : spsDCVoltageSourceLib/DC Voltage Source  Amplitude=100  Measurements=None
  NOT{,1..3} (4 alike) : Logic  Operator=NOT  AllPortsSameDT=off  OutDataTypeStr=boolean
  Relational Operator4 : RelationalOperator  OutDataTypeStr=boolean  InputSameDT=off
  Relational Operator5 : RelationalOperator  Operator=<=  OutDataTypeStr=boolean  InputSameDT=off
  Relational Operator6 : RelationalOperator  Operator=<=  OutDataTypeStr=boolean  InputSameDT=off
  Relational Operator7 : RelationalOperator  OutDataTypeStr=boolean  InputSameDT=off
  Repeating Sequence1 : simulink/Sources/Repeating Sequence  rep_seq_t=[0 0.00025 0.0005 0.00075 0.001]*(1/fr)*(1/fc)*(1/2)  rep_seq_y="[0 1 0 -1 0  ]"
  Repeating Sequence2 : simulink/Sources/Repeating Sequence  rep_seq_t=[0 0.00025 0.0005 0.00075 0.001]*(1/fr)*(1/fc)*(1/2)  rep_seq_y=[ 0 -1 0 1 0 ]
  Repeating Sequence5 : simulink/Sources/Repeating Sequence  rep_seq_t=[0 0.00025 0.0005 0.00075 0.001]*(1/fr)*(1/fc)*(1/2)  rep_seq_y=[1 0 -1 0 1]
  Repeating Sequence7 : simulink/Sources/Repeating Sequence  rep_seq_t=[0 0.00025 0.0005 0.00075 0.001]*(1/fr)*(1/fc)*(1/2)  rep_seq_y=[-1 0 1 0 -1]
  SW{1..8} (8 alike) : spsIGBTDiodeLib/IGBT//Diode  Ron=1e-3  Rs=1e5  Cs=inf  Measurements=on
  Sine Wave1 : Sin  Amplitude=Ma  Frequency=2*pi*fr  Phase=ph  SampleTime=0
  Sine Wave2 : Sin  Amplitude=Ma  Frequency=2*pi*fr  Phase=ph  SampleTime=0
  Va : PMIOPort  Tag=PMCPort  Side=Right
  N : PMIOPort  Tag=PMCPort  Port=2  Side=Right
  wires:
  Sine Wave2/1 -> Relational Operator4/1, Relational Operator6/1
  Repeating Sequence1/1 -> Relational Operator4/2
  Repeating Sequence2/1 -> Relational Operator6/2
  Relational Operator4/1 -> NOT/1, [S1]
  NOT/1 -> [S3]
  NOT1/1 -> [S4]
  Relational Operator6/1 -> [S2], NOT1/1
  Repeating Sequence7/1 -> Relational Operator7/2
  Repeating Sequence5/1 -> Relational Operator5/2
  Sine Wave1/1 -> Relational Operator7/1, Relational Operator5/1
  Relational Operator5/1 -> [S6], NOT3/1
  Relational Operator7/1 -> [S5], NOT2/1
  NOT2/1 -> [S7]
  NOT3/1 -> [S8]
  [S3] -> SW3/1
  [S4] -> SW4/1
  [S6] -> SW6/1
  [S5] -> SW5/1
  [S7] -> SW7/1
  [S8] -> SW8/1
  [S1] -> SW1/1
  [S2] -> SW2/1
  connections:
  SW2/RConn1 -- Va/RConn1
  SW4/RConn1 -- 100V/LConn1 -- SW3/RConn1
  SW8/RConn1 -- 100V1/LConn1 -- SW7/RConn1
  SW1/RConn1 -- SW3/LConn1 -- SW6/RConn1 -- SW8/LConn1
  SW5/LConn1 -- 100V1/RConn1 -- SW6/LConn1
  N/RConn1 -- SW5/RConn1 -- SW7/LConn1
  100V/RConn1 -- SW1/LConn1 -- SW2/LConn1
